simulink library "IMT_Library"  (R2020b)
settings: Solver=VariableStepAuto  StartTime=0.0  StopTime=10.0  RelTol=1e-3
libraries: slpidlib x1, simulink_extras x1
settings Model: Creator=Mr_Li  LastModifiedBy=Mr_Li

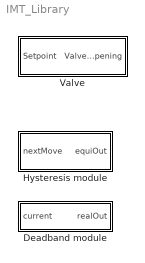
== system IMT_Library ==
  Deadband module : Subsystem  mask{upper=0, lower=0}
      mask prompts: upper "Upper limit"; lower "Lower limit"
  Hysteresis module : Subsystem  mask{hysteresisSize=0}
      mask prompts: hysteresisSize "Hysteresis loop wide"
  Valve : Subsystem  mask{upper=101, lower=1.2, movementThreshold=1}
      mask prompts: upper "Valve upper opening(%)"; lower "Valve lower opening(%)"; movementThreshold "Valve movement threshold"

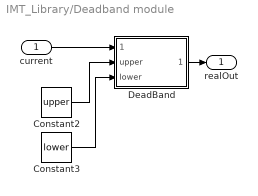
== system IMT_Library/Deadband module ==
  current : Inport
  Constant2 : Constant  Value=upper
  Constant3 : Constant  Value=lower
  DeadBand : MATLAB Function  TreatAsAtomicUnit=on
  realOut : Outport
  wires:
  DeadBand/1(realOut) -> realOut/1
  current/1 -> DeadBand/1(current)
  Constant3/1 -> DeadBand/3(lower)
  Constant2/1 -> DeadBand/2(upper)

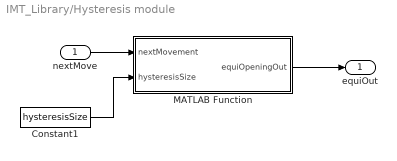
== system IMT_Library/Hysteresis module ==
  nextMove : Inport
  Constant1 : Constant  Value=hysteresisSize
  MATLAB Function : MATLAB Function  TreatAsAtomicUnit=on
  equiOut : Outport
  wires:
  nextMove/1 -> MATLAB Function/1(nextMovement)
  MATLAB Function/1(equiOpeningOut) -> equiOut/1
  Constant1/1 -> MATLAB Function/2(hysteresisSize)

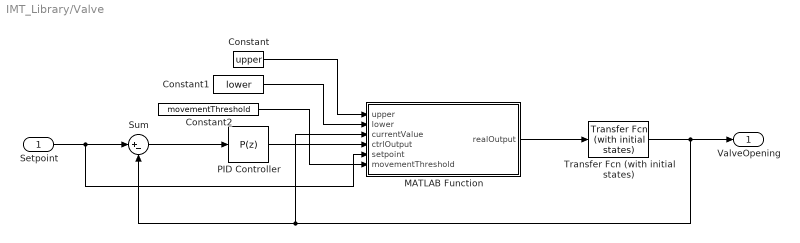
== system IMT_Library/Valve ==
  Setpoint : Inport
  Constant : Constant  Value=upper
  Constant1 : Constant  Value=lower
  Constant2 : Constant  Value=movementThreshold
  MATLAB Function : MATLAB Function  TreatAsAtomicUnit=on
  PID Controller : slpidlib/PID Controller  Controller=P  Form=Parallel  TimeDomain=Discrete-time  UseExternalTs=off  SampleTime=-1  IntegratorMethod=Forward Euler  FilterMethod=Forward Euler  ControllerParametersSource=internal  P=1  I=1  D=0  UseFilter=on  N=100  TunerSelectOption=Transfer Function Based (PID Tuner App)  InitialConditionSource=internal  InitialConditionForIntegrator=0  InitialConditionForFilter=0  DifferentiatorICPrevScaledInput=0  ExternalReset=none  TrackingMode=off  Kt=1  LimitOutput=on  SatLimitsSource=internal  UpperSaturationLimit=0.693  LowerSaturationLimit=-0.693  LinearizeAsGain=on  AntiWindupMode=none  Kb=1  POutMin=[]  POutMax=[]  IOutMin=[]  IOutMax=[]  DOutMin=[]  DOutMax=[]  NOutMin=[]  NOutMax=[]  SumOutMin=[]  SumOutMax=[]  SaturationOutMin=[]  SaturationOutMax=[]  PParamMin=[]  PParamMax=[]  IParamMin=[]  IParamMax=[]  DParamMin=[]  DParamMax=[]  NParamMin=[]  NParamMax=[]  KbParamMin=[]  KbParamMax=[]  KtParamMin=[]  KtParamMax=[]  KbOutMin=[]  KbOutMax=[]  KtOutMin=[]  KtOutMax=[]  IntegratorOutMin=[]  IntegratorOutMax=[]  FilterOutMin=[]  FilterOutMax=[]  SumI1OutMin=[]  SumI1OutMax=[]  SumI2OutMin=[]  SumI2OutMax=[]  SumI3OutMin=[]  SumI3OutMax=[]  SumI4OutMin=[]  SumI4OutMax=[]  SumDOutMin=[]  SumDOutMax=[]  DifferentiatorOutMin=[]  DifferentiatorOutMax=[]  FilterDiffOutCoefMin=[]  FilterDiffOutCoefMax=[]  ReciprocalOutMin=[]  ReciprocalOutMax=[]  SumDenOutMin=[]  SumDenOutMax=[]  SumNumOutMin=[]  SumNumOutMax=[]  DivideOutMin=[]  DivideOutMax=[]  UdiffTsProdOutMin=[]  UdiffTsProdOutMax=[]  NTsProdOutMin=[]  NTsProdOutMax=[]  UintegralTsProdOutMin=[]  UintegralTsProdOutMax=[]  UngainTsProdOutMin=[]  UngainTsProdOutMax=[]  IntegratorContinuousStateAttributes=''  IntegratorStateMustResolveToSignalObject=off  IntegratorRTWStateStorageClass=Auto  FilterContinuousStateAttributes=''  FilterStateMustResolveToSignalObject=off  FilterRTWStateStorageClass=Auto  ParallelPVariant=InternalParameters  IdealPVariant=Disabled  IVariant=Disabled  DVariant=Disabled  IntegratorVariant=Disabled  SatVariant=Enabled  AWVariant=Disabled  PCopyVariant=Disabled  TRVariant=Disabled  FdbkBlocksVariant=Forward  IdealPFdbkVariant=Disabled  SatFdbkVariant=Disabled  DerivativeFilterVariant=Disabled  NVariant=Disabled  NCopyVariant=Disabled_SignalSpec  FilterICVariant=Disabled  IntegratorICVariant=Disabled  ExternalResetVariant=Disabled  TRSumVariant=Passthrough  SumFdbkVariant=Disabled  SumVariant=Passthrough_P  TsampFilterVariant=InternalTs  TsampNgainVariant=Passthrough  TsampIntegralVariant=Disabled_SignalSpec  ExternalSaturationOutDataTypeStr=Inherit: Same as second input
  Sum : Sum  Inputs=|+-
  Transfer Fcn (with initial states) : simulink_extras/Additional Linear/Transfer Fcn (with initial states)  N=[1]  D="[1  0]"  X0=1.2
  ValveOpening : Outport
  wires:
  MATLAB Function/1(realOutput) -> Transfer Fcn (with initial states)/1
  Constant1/1 -> MATLAB Function/2(lower)
  Sum/1 -> PID Controller/1
  Transfer Fcn (with initial states)/1 -> ValveOpening/1, Sum/2, MATLAB Function/3(currentValue)
  Constant/1 -> MATLAB Function/1(upper)
  Constant2/1 -> MATLAB Function/6(movementThreshold)
  Setpoint/1 -> MATLAB Function/5(setpoint), Sum/1
  PID Controller/1 -> MATLAB Function/4(ctrlOutput)

== matlab function IMT_Library/Hysteresis module/MATLAB Function ==
  settings: updateMethod=DISCRETE
  data: nextMovement input; equiOpeningOut output; hysteresisSize input
function equiOpeningOut  = fcn(nextMovement,hysteresisSize)
%[equiOpeningOut,previousDirectionOut]
persistent previousDirection; %阀门移动是否同向,默认true为上升
persistent hysteresisBuffer;
persistent equiOpening; %阀门等效开度，带缓存
persistent currentValve; %缓存上一步的阀门开度，实际的阀门开度

% 静态变量初始化
if(isempty(currentValve))
    currentValve=nextMovement;
end

if(isempty(equiOpening))
    equiOpening=nextMovement;
end

if(isempty(previousDirection))
    previousDirection=true;
%     previousDirectionOut=previousDirection;
    hysteresisBuffer=hysteresisSize;
end

if(nextMovement==currentValve)
    equiOpeningOut=equiOpening;
%     previousDirectionOut=previousDirection;
    return;
end

% 判断阀门运动方向
if(((nextMovement-currentValve)>=0)~=previousDirection)
    if(abs(currentValve-nextMovement)>0.1)
        %避免等效下降速度快于实际，而产生的方向误改变情况
        previousDirection=((nextMovement-currentValve)>=0);%equiOpening
%         previousDirectionOut=previousDirection;
        hysteresisBuffer=hysteresisSize;
    end
%     previousDirectionOut=previousDirection;
end

% 计算实际阀门增量和buffer
hysteresisBuffer=hysteresisBuffer-abs(currentValve-nextMovement);


% 计算buffer后的
if(hysteresisBuffer<=0)
%     表明抵消完buffer或者抵消完buffer后还有多余增量
    if(previousDirection)% 为什么没有三目表达式
        equiOpening=equiOpening+abs(hysteresisBuffer);
        equiOpeningOut=equiOpening;
        currentValve=nextMovement;
    else
        equiOpening=equiOpening+abs(hysteresisBuffer)*(-1);
        equiOpeningOut=equiOpening;
        currentValve=nextMovement;
    end
%     previousDirectionOut=previousDirection;
    hysteresisBuffer=0;
else
%     equiOpening=currentValve;
    equiOpeningOut=equiOpening;
    currentValve=nextMovement;
%     previousDirectionOut=previousDirection;
end

== matlab function IMT_Library/Valve/MATLAB Function ==
  settings: updateMethod=DISCRETE
  data: upper input; realOutput output; lower input; currentValue input; ctrlOutput input; setpoint input; movementThreshold input
function realOutput = fcn(upper,lower,currentValue,ctrlOutput,setpoint,movementThreshold)

if(currentValue>setpoint)
    if(currentValue<lower)
        realOutput=0;
     elseif(abs(currentValue-setpoint)<movementThreshold)
        realOutput=0;
    else
        realOutput=ctrlOutput;
    end
else
    if(currentValue>upper)
        realOutput=0;
    
    else
        realOutput=ctrlOutput;
    end
end
    
% if(abs(currentValue-setpoint)<1.2)
%     if(currentValue>setpoint)
%         realOutput=0;
%     elseif((currentValue)<lower)
%         realOutput=0;
%     else
%         realOutput=ctrlOutput;
%     end
% end

== matlab function IMT_Library/Deadband module/DeadBand ==
  settings: updateMethod=CONTINUOUS
  data: current input; upper input; realOut output; lower input
function realOut = deadBandLimit(current,upper,lower)
if(current<=lower)
    realOut = 0;
elseif(current>upper)
    realOut=upper;
else
    realOut=current;
end
